simulink model "arduino_wifiudpsend"  (R2018b)
settings: Solver=ode3  StartTime=0.0  StopTime=inf  FixedStep=1  RelTol=1e-3  EnableMultiTasking=on
libraries: xpcutilitieslib x1, simulink x1, arduinowifilib x1
settings Model: ExtModeTrigDuration=2  Creator=The MathWorks, Inc.  LastModifiedBy=Boreth
settings DataIOCC: LimitDataPoints=on  SaveOutput=off  SaveState=on
settings OptimizationCC: LifeSpan=1  MaxStackSize=64
settings DebuggingCC: UnderspecifiedInitializationDetection=Classic  MergeDetectMultiDrivingBlocksExec=none  AllowSymbolicDim=off  LibraryContextMissingDiagnostic=none  SFUnexpectedBacktrackingDiag=warning  SFNoUnconditionalDefaultTransitionDiag=warning  SFExecutionAtInitializationDiag=none
settings HardwareCC: ProdBitPerInt=16  ProdBitPerPointer=16  ProdBitPerSizeT=16  ProdBitPerPtrDiffT=16  ProdLargestAtomicFloat=None  ProdWordSize=8  ProdHWDeviceType=Atmel->AVR  UseEmbeddedCoderFeatures=off  UseSimulinkCoderFeatures=off
settings ModelReferenceCC: PropagateSignalLabelsOutOfModel=off
settings SFSimCC: SimUseLocalCustomCode=off  MATLABDynamicMemAlloc=off
settings RTWCC: SystemTargetFile=ert.tlc  HardwareBoard=Arduino Mega 2560  TemplateMakefile=ert_default_tmf  GenerateReport=on  RTWVerbose=off  RTWUseLocalCustomCode=off  Toolchain=Arduino AVR  BuildConfiguration=Faster Runs  LaunchReport=on
settings CodeAppCC: ForceParamTrailComments=on  OperatorAnnotations=on  StateflowObjectComments=on  MATLABSourceComments=on
settings ERTTargetCC: MultiwordLength=2048  ERTCustomFileBanners=off  SupportContinuousTime=on  SupportNonInlinedSFcns=on  RemoveResetFunc=off  SupportVariableSizeSignals=on  ModelStepFunctionPrototypeControlCompliant=off
settings ConfigComp: CovMetricSettings=dw  CovHtmlReporting=on  CovSaveCumulativeToWorkspaceVar=on  CovSaveSingleToWorkspaceVar=on  CovExternalEMLEnable=off  CovSFcnEnable=off

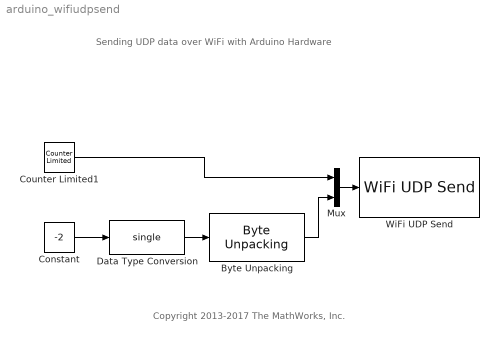
== system arduino_wifiudpsend ==
  note: Sending UDP data over WiFi
      |  with Arduino Hardware
  note: Copyright 2013-2017 The MathWorks, Inc.
  "Byte Unpacking " : xpcutilitieslib/Byte Unpacking   MaskUnpackedDataTypes={'uint8'}  MaskUnpackedDataSizes={[4]}  MaskAlignment=1
      settings: SourceProductName=Simulink Real-Time  SourceProductBaseCode=XP
  Constant : Constant  Value=-2
  Counter Limited1 : simulink/Sources/Counter Limited  uplimit=10  tsamp=1
  Data Type Conversion : DataTypeConversion  OutDataTypeStr=single
  Mux : Mux  Inputs=2
  WiFi UDP Send : arduinowifilib/WiFi UDP Send  remoteIPOctetString=192.168.1.251  remoteport=50002  localport=50001  remoteipoctet1=192  remoteipoctet2=168  remoteipoctet3=1  remoteipoctet4=251  wifiUDPIndex=0  blockPlatform=arduino  isARMArch=false
      settings: SourceProductName=Simulink Support Package for Arduino Hardware  SourceProductBaseCode=ARDUINO
  wires:
  Constant/1 -> Data Type Conversion/1
  Counter Limited1/1 -> Mux/1
  Data Type Conversion/1 -> "Byte Unpacking "/1
  Mux/1 -> WiFi UDP Send/1
  "Byte Unpacking "/1 -> Mux/2
